simulink model "gm_hdl_model_fixed_vnl"  (R2024a)
settings: Solver=FixedStepDiscrete  StartTime=0.0  StopTime=SIM_TIME  RelTol=1e-3
undefined symbols (not defined in the file or in its folder): a, b, BUFFER_LEN, c, SAMPLING_FREQ, signal_1
libraries: hdlsllib x41, simulink x16, dspsigops x15, simulink_extras x5, dsphdlxfrm2 x2, dspsrcs4 x1
(part 1 of 3)
settings Model: SimulationMode=accelerator  Creator=Jan Rosa  LastModifiedBy=Jan Rosa
settings OptimizationCC: BlockReduction=off  ConditionallyExecuteInputs=off  DefaultParameterBehavior=Inlined  InheritOutputTypeSmallerThanSingle=on
settings DebuggingCC: SignalRangeChecking=warning  AlgebraicLoopMsg=error  SolverPrmCheckMsg=warning  InheritedTsInSrcMsg=none  SingleTaskRateTransMsg=error  UnderSpecifiedDataTypeMsg=warning  UnconnectedInputMsg=error  UnconnectedOutputMsg=error  UnconnectedLineMsg=error  ModelReferenceVersionMismatchMessage=warning  ModelReferenceIOMismatchMessage=warning  ModelReferenceNoExplicitFinalValueMsg=warning  StateNameClashWarn=warning
settings HardwareCC: ProdBitPerPointer=32  ProdBitPerSizeT=32  ProdBitPerPtrDiffT=32  ProdLargestAtomicFloat=None  ProdIntDivRoundTo=Undefined  ProdEndianess=Unspecified  ProdWordSize=32  ProdHWDeviceType=ASIC/FPGA->ASIC/FPGA  TargetBitPerPointer=64  TargetBitPerSizeT=64  TargetBitPerPtrDiffT=64  TargetLongLongMode=on  TargetIntDivRoundTo=Zero  TargetEndianess=LittleEndian  TargetWordSize=64  TargetHWDeviceType=Custom Processor->MATLAB Host Computer  ProdEqTarget=off
settings ModelReferenceCC: EnableRefExpFcnMdlSchedulingChecks=on  EnableParallelModelReferenceBuilds=on

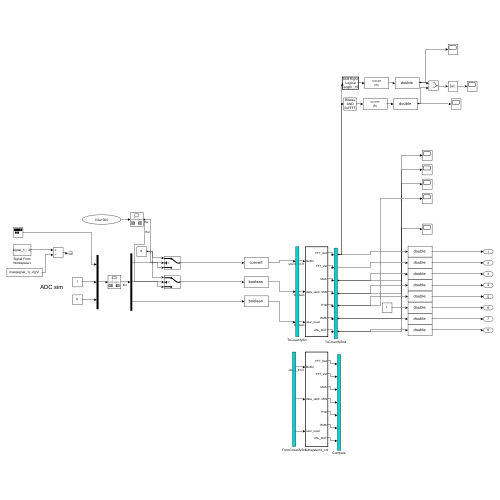
[thumbnail: Simulink's stored preview of the top-level diagram]
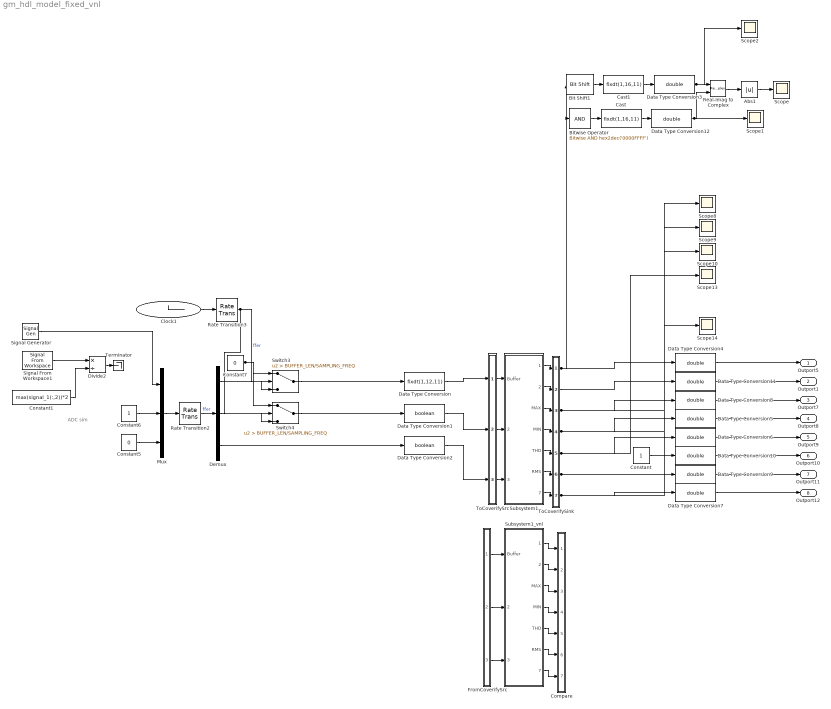
== system gm_hdl_model_fixed_vnl ==
  note: ADC sim
  Abs1 : Abs  SaturateOnIntegerOverflow=off
  Bit Shift1 : hdlsllib/Logic and Bit Operations/Bit Shift  mode=Shift Right Logical  N=16
  Bitwise Operator : simulink/Logic and Bit Operations/Bitwise Operator  logicop=AND  UseBitMask=on  BitMask=hex2dec('0000FFFF')  BitMaskRealWorld=Stored Integer
  Cast : DataTypeConversion  OutDataTypeStr=fixdt(1,16,11)  ConvertRealWorld=Stored Integer (SI)  SaturateOnIntegerOverflow=off  RndMeth=Floor
  Cast1 : DataTypeConversion  OutDataTypeStr=fixdt(1,16,11)  ConvertRealWorld=Stored Integer (SI)  SaturateOnIntegerOverflow=off  RndMeth=Floor
  Clock1 : Clock
  Compare : Subsystem
      mask Display: disp('')
  Constant : Constant
  Constant1 : Constant  Value=max(signal_1(:,2))*2
  Constant5 : Constant  Value=0
  Constant6 : Constant
  Constant7 : Constant  Value=0  SampleTime=1/SAMPLING_FREQ
  Data Type Conversion : DataTypeConversion  OutDataTypeStr=fixdt(1,12,11)  SaturateOnIntegerOverflow=off  RndMeth=Floor  LockScale=on
  Data Type Conversion1 : DataTypeConversion  OutDataTypeStr=boolean  SaturateOnIntegerOverflow=off  RndMeth=Floor  LockScale=on
  Data Type Conversion{3..12} (10 alike) : DataTypeConversion  OutDataTypeStr=double  SaturateOnIntegerOverflow=off  RndMeth=Floor
  Data Type Conversion2 : DataTypeConversion  OutDataTypeStr=boolean  SaturateOnIntegerOverflow=off  RndMeth=Floor  LockScale=on
  Demux : Demux  Outputs=3
  Divide2 : Product  Inputs=*/
  FromCoverifySrc : Subsystem
      mask Display: disp('')
  Mux : Mux  Inputs=3
  Rate Transition2 : RateTransition  Integrity=off  Deterministic=off  OutPortSampleTime=1/SAMPLING_FREQ
  Rate Transition3 : RateTransition  Integrity=off  Deterministic=off  OutPortSampleTime=1/SAMPLING_FREQ
  Real-Imag to Complex : RealImagToComplex
  Scope{,1..2,8..10,13..14} (8 alike) : Scope
  Signal Generator : SignalGenerator  WaveForm=square  Amplitude=0.49999  Frequency=SAMPLING_FREQ/(16*16)
  Signal From Workspace1 : dspsrcs4/Signal From Workspace  X=signal_1(:, 2)  Ts=signal_1(2, 1)  nsamps=1  OutputAfterFinalValue=Cyclic repetition  ignoreOrWarnInputAndFrameLengths=off  OutputFrames=off
  Subsystem1 : Subsystem  TreatAsAtomicUnit=on
  Subsystem1_vnl : Subsystem  TreatAsAtomicUnit=on
  Switch3 : Switch  Criteria=u2 > Threshold  Threshold=BUFFER_LEN/SAMPLING_FREQ  SaturateOnIntegerOverflow=off  InputSameDT=off
  Switch4 : Switch  Criteria=u2 > Threshold  Threshold=BUFFER_LEN/SAMPLING_FREQ  SaturateOnIntegerOverflow=off  InputSameDT=off
  Terminator : Terminator
  ToCoverifySink : Subsystem
      mask Display: disp('')
  ToCoverifySrc : Subsystem
      mask Display: disp('')
  Outport5 : Outport
  Outport1 : Outport  Port=2
  Outport7 : Outport  Port=3
  Outport8 : Outport  Port=4
  Outport9 : Outport  Port=5
  Outport10 : Outport  Port=6
  Outport11 : Outport  Port=7
  Outport12 : Outport  Port=8
  wires:
  Switch4/1 -> Data Type Conversion1/1
  Constant7/1 -> Switch4/1, Switch3/1
  Rate Transition3/1 -> Switch4/2, Switch3/2  "ffer"
  Demux/2 -> Switch4/3
  Clock1/1 -> Rate Transition3/1
  Demux/3 -> Data Type Conversion2/1
  Switch3/1 -> Data Type Conversion/1
  Demux/1 -> Switch3/3
  Mux/1 -> Rate Transition2/1
  Abs1/1 -> Scope/1
  Rate Transition2/1 -> Demux/1  "ffer"
  Constant5/1 -> Mux/3
  Signal From Workspace1/1 -> Divide2/1
  Constant6/1 -> Mux/2
  Constant1/1 -> Divide2/2
  Data Type Conversion4/1 -> Outport5/1
  Data Type Conversion8/1 -> Outport7/1
  Data Type Conversion5/1 -> Outport8/1
  Data Type Conversion6/1 -> Outport9/1
  Data Type Conversion10/1 -> Outport10/1
  Data Type Conversion7/1 -> Outport12/1
  Data Type Conversion9/1 -> Outport11/1
  Data Type Conversion11/1 -> Outport1/1
  Data Type Conversion3/1 -> Scope2/1, Real-Imag to Complex/1
  Real-Imag to Complex/1 -> Abs1/1
  Signal Generator/1 -> Mux/1
  Bit Shift1/1 -> Cast1/1
  Bitwise Operator/1 -> Cast/1
  Data Type Conversion12/1 -> Scope1/1, Real-Imag to Complex/2
  Cast/1 -> Data Type Conversion12/1
  Cast1/1 -> Data Type Conversion3/1
  Constant/1 -> Data Type Conversion10/1
  Divide2/1 -> Terminator/1
  ToCoverifySrc/1(out1) -> Subsystem1/1(Buffer)
  ToCoverifySrc/2(out2) -> Subsystem1/2(data_valid)
  ToCoverifySrc/3(out3) -> Subsystem1/3(user_reset)
  Subsystem1/1(FFT_Dat) -> ToCoverifySink/1(in1)
  Subsystem1/2(FFT_Val) -> ToCoverifySink/2(in2)
  Subsystem1/3(MAX) -> ToCoverifySink/3(in3)
  Subsystem1/4(MIN) -> ToCoverifySink/4(in4)
  Subsystem1/5(THD) -> ToCoverifySink/5(in5)
  Subsystem1/6(RMS) -> ToCoverifySink/6(in6)
  Subsystem1/7(VAL_OUT) -> ToCoverifySink/7(in7)
  Data Type Conversion/1 -> ToCoverifySrc/1(in1)
  Data Type Conversion1/1 -> ToCoverifySrc/2(in2)
  Data Type Conversion2/1 -> ToCoverifySrc/3(in3)
  ToCoverifySink/1(out1) -> Bit Shift1/1, Bitwise Operator/1, Data Type Conversion4/1
  ToCoverifySink/2(out2) -> Data Type Conversion11/1
  ToCoverifySink/3(out3) -> Scope10/1, Data Type Conversion8/1
  ToCoverifySink/4(out4) -> Scope9/1, Data Type Conversion5/1
  ToCoverifySink/5(out5) -> Scope13/1, Data Type Conversion6/1
  ToCoverifySink/6(out6) -> Scope8/1, Data Type Conversion9/1
  ToCoverifySink/7(out7) -> Scope14/1, Data Type Conversion7/1
  FromCoverifySrc/1(out1) -> Subsystem1_vnl/1(Buffer)
  FromCoverifySrc/2(out2) -> Subsystem1_vnl/2(data_valid)
  FromCoverifySrc/3(out3) -> Subsystem1_vnl/3(user_reset)
  Subsystem1_vnl/1(FFT_Dat) -> Compare/1(in1)
  Subsystem1_vnl/2(FFT_Val) -> Compare/2(in2)
  Subsystem1_vnl/3(MAX) -> Compare/3(in3)
  Subsystem1_vnl/4(MIN) -> Compare/4(in4)
  Subsystem1_vnl/5(THD) -> Compare/5(in5)
  Subsystem1_vnl/6(RMS) -> Compare/6(in6)
  Subsystem1_vnl/7(VAL_OUT) -> Compare/7(in7)

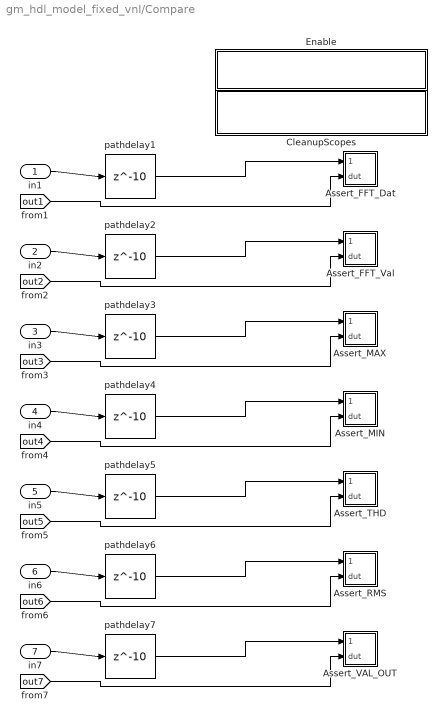
== system gm_hdl_model_fixed_vnl/Compare ==
  in1 : Inport
  in2 : Inport  Port=2
  in3 : Inport  Port=3
  in4 : Inport  Port=4
  in5 : Inport  Port=5
  in6 : Inport  Port=6
  in7 : Inport  Port=7
  Assert_FFT_Dat : Subsystem
      settings: LibrarySourceBlock=hdlmdlgenlib/AssertEqIDC
  Assert_FFT_Val : Subsystem
      settings: LibrarySourceBlock=hdlmdlgenlib/AssertEqIDC
  Assert_MAX : Subsystem
      settings: LibrarySourceBlock=hdlmdlgenlib/AssertEqIDC
  Assert_MIN : Subsystem
      settings: LibrarySourceBlock=hdlmdlgenlib/AssertEqIDC
  Assert_RMS : Subsystem
      settings: LibrarySourceBlock=hdlmdlgenlib/AssertEqIDC
  Assert_THD : Subsystem
      settings: LibrarySourceBlock=hdlmdlgenlib/AssertEqIDC
  Assert_VAL_OUT : Subsystem
      settings: LibrarySourceBlock=hdlmdlgenlib/AssertEqIDC
  CleanupScopes : Subsystem
      settings: OpenFcn=|
      | blkName = gcb; %self block
      | idx = regexp(blkName, '/CleanupScopes$', 'once');
      | blkParent = blkName(1:idx-1);
      | blks=find_system(blkParent, 'LookUnderMasks', 'all','blocktype', 'Scope');
      | for itr = 1:length(blks)
      | 	 hScopeCfg = get_param(blks{itr},'ScopeConfiguration');
      | 	 hScopeCfg.Visible = ~ hScopeCfg.Visible;
      | end
      | drawnow;
      mask Display: fprintf(message('hdlcoder:cosim:vnl_dblclick').getString());
  Enable : Subsystem
      settings: OpenFcn=|
      | blkName = gcb;
      | idx = regexp(blkName, '/Enable$', 'once');
      | blkParent = blkName(1:idx-1);
      | blks=find_system(blkParent, 'LookUnderMasks', 'all','blocktype', 'Assertion');
      | e = get_param(blks{1}, 'Enabled');
      | if strcmp(e, 'on'), f= 'off';, else, f = 'on';, end
      | for ii=1:length(blks), set_param(blks{ii}, 'Enabled', f);, end
      | set_param(gcb, 'MaskDisplay',['fprintf(message(''hdlcoder:cosim:vnl_dblclick_assertions'',','''',upper(e),'''',').getString())']);
      mask Display: fprintf(message('hdlcoder:cosim:vnl_dblclick_assertions','OFF').getString());
  pathdelay{1..7} (7 alike) : Delay  DelayLength=10
  wires:
  in1/1 -> pathdelay1/1
  pathdelay1/1 -> Assert_FFT_Dat/1(cosim)
  [out1] -> Assert_FFT_Dat/2(dut)
  in2/1 -> pathdelay2/1
  pathdelay2/1 -> Assert_FFT_Val/1(cosim)
  [out2] -> Assert_FFT_Val/2(dut)
  in3/1 -> pathdelay3/1
  pathdelay3/1 -> Assert_MAX/1(cosim)
  [out3] -> Assert_MAX/2(dut)
  in4/1 -> pathdelay4/1
  pathdelay4/1 -> Assert_MIN/1(cosim)
  [out4] -> Assert_MIN/2(dut)
  in5/1 -> pathdelay5/1
  pathdelay5/1 -> Assert_THD/1(cosim)
  [out5] -> Assert_THD/2(dut)
  in6/1 -> pathdelay6/1
  pathdelay6/1 -> Assert_RMS/1(cosim)
  [out6] -> Assert_RMS/2(dut)
  in7/1 -> pathdelay7/1
  pathdelay7/1 -> Assert_VAL_OUT/1(cosim)
  [out7] -> Assert_VAL_OUT/2(dut)

== system gm_hdl_model_fixed_vnl/FromCoverifySrc ==
  out1 : Outport
  out2 : Outport  Port=2
  out3 : Outport  Port=3
  wires:
  [in1] -> out1/1
  [in2] -> out2/1
  [in3] -> out3/1

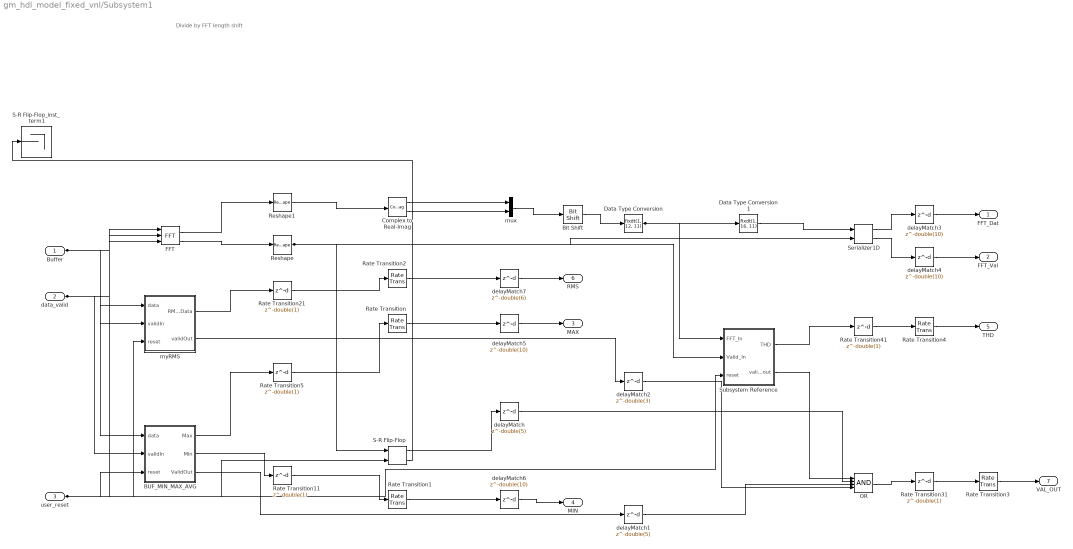
== system gm_hdl_model_fixed_vnl/Subsystem1 ==
  note: Divide by FFT length shift
  Buffer : Inport  OutDataTypeStr=fixdt(1, 12, 11)  PortDimensions=1  SampleTime=1e-08
  data_valid : Inport  Port=2  OutDataTypeStr=boolean  PortDimensions=1  SampleTime=1e-08
  user_reset : Inport  Port=3  OutDataTypeStr=boolean  PortDimensions=1  SampleTime=1e-08
  BUF_MIN_MAX_AVG : Subsystem
  Bit Shift : hdlsllib/Logic and Bit Operations/Bit Shift  mode=Shift Right Arithmetic  N=double(11)
  Complex to Real-Imag : ComplexToRealImag  SampleTime=1e-08
  Data Type Conversion : DataTypeConversion  OutDataTypeStr=fixdt(1, 12, 11)  SampleTime=1e-08  SaturateOnIntegerOverflow=off  RndMeth=Floor
  Data Type Conversion1 : DataTypeConversion  OutDataTypeStr=fixdt(1, 16, 11)  SampleTime=1e-08  SaturateOnIntegerOverflow=off  RndMeth=Floor
  FFT : dsphdlxfrm2/FFT  Architecture=Streaming Radix 2^2  FFTLengthSource=Property  FFTLength=BUFFER_LEN  FFTLengthMax=1024  ComplexMultiplication=Use 4 multipliers and 2 adders  BitReversedOutput=off  BitReversedInput=off  Normalize=off  SimulateUsing=Code generation  RoundingMethod=Floor  ResetInputPort=on  StartOutputPort=off  EndOutputPort=off
  OR : Logic  Inputs=4  AllPortsSameDT=off  OutDataTypeStr=boolean  SampleTime=1e-08
  Rate Transition : RateTransition  Integrity=off  Deterministic=off  InitialCondition="fi(0,0,16,16,\"hex\",\"0000\")"  OutPortSampleTimeOpt=Multiple of input port sample time  OutPortSampleTimeMultiple=1/2
  Rate Transition1 : RateTransition  Integrity=off  Deterministic=off  InitialCondition="fi(0,1,16,15,\"hex\",\"0000\")"  OutPortSampleTimeOpt=Multiple of input port sample time  OutPortSampleTimeMultiple=1/2
  Rate Transition{5,11,21,31,41} (5 alike) : Delay  DelayLength=double(1)  InitialCondition=0  SampleTime=1e-08
  Rate Transition2 : RateTransition  Integrity=off  Deterministic=off  InitialCondition="fi(0,0,16,7,\"hex\",\"0000\")"  OutPortSampleTimeOpt=Multiple of input port sample time  OutPortSampleTimeMultiple=1/2
  Rate Transition3 : RateTransition  Integrity=off  Deterministic=off  OutPortSampleTimeOpt=Multiple of input port sample time  OutPortSampleTimeMultiple=1/2
  Rate Transition4 : RateTransition  Integrity=off  Deterministic=off  InitialCondition="fi(0,1,18,10,\"hex\",\"00000\")"  OutPortSampleTimeOpt=Multiple of input port sample time  OutPortSampleTimeMultiple=1/2
  Reshape : Reshape
  Reshape1 : Reshape
  S-R Flip-Flop : simulink_extras/Flip Flops/S-R Flip-Flop  initial_condition=0
  S-R Flip-Flop_inst_term1 : Terminator
  Serializer1D : hdlsllib/HDL Operations/Serializer1D  Ratio=2  IdleCycles=0  validIn=on  startOut=off  validOut=on  inputDataDimensions=2  inputSampleTime=1e-08  inputSignalType=real
  Subsystem Reference : Subsystem
  delayMatch : Delay  DelayLength=double(5)  InitialCondition=0  SampleTime=1e-08
  delayMatch1 : Delay  DelayLength=double(5)  InitialCondition=0  SampleTime=1e-08
  delayMatch2 : Delay  DelayLength=double(3)  InitialCondition=0  SampleTime=1e-08
  delayMatch{3..6} (4 alike) : Delay  DelayLength=double(10)  InitialCondition=0  SampleTime=5e-09
  delayMatch7 : Delay  DelayLength=double(6)  InitialCondition=0  SampleTime=5e-09
  mux : Mux  Inputs=2
  myRMS : Subsystem
  FFT_Dat : Outport  SampleTime=5e-09
  FFT_Val : Outport  Port=2  SampleTime=5e-09
  MAX : Outport  Port=3  SampleTime=5e-09
  MIN : Outport  Port=4  SampleTime=5e-09
  THD : Outport  Port=5  SampleTime=5e-09
  RMS : Outport  Port=6  SampleTime=5e-09
  VAL_OUT : Outport  Port=7  SampleTime=5e-09
  wires:
  Rate Transition2/1 -> delayMatch7/1
  Rate Transition1/1 -> delayMatch6/1
  Rate Transition/1 -> delayMatch5/1
  Serializer1D/2 -> delayMatch4/1
  Serializer1D/1 -> delayMatch3/1
  myRMS/2(validOut) -> delayMatch2/1
  BUF_MIN_MAX_AVG/3(ValidOut) -> delayMatch1/1
  S-R Flip-Flop/1 -> delayMatch/1
  OR/1 -> Rate Transition31/1
  Data Type Conversion1/1 -> Serializer1D/1
  Bit Shift/1 -> Data Type Conversion/1
  mux/1 -> Bit Shift/1
  Complex to Real-Imag/2 -> mux/2
  Complex to Real-Imag/1 -> mux/1
  Reshape1/1 -> Complex to Real-Imag/1
  S-R Flip-Flop/2 -> S-R Flip-Flop_inst_term1/1
  Rate Transition41/1 -> Rate Transition4/1
  Rate Transition31/1 -> Rate Transition3/1
  Rate Transition21/1 -> Rate Transition2/1
  Rate Transition11/1 -> Rate Transition1/1
  Rate Transition5/1 -> Rate Transition/1
  delayMatch/1 -> OR/2
  delayMatch4/1 -> FFT_Val/1
  Rate Transition4/1 -> THD/1
  Rate Transition3/1 -> VAL_OUT/1
  delayMatch7/1 -> RMS/1
  delayMatch6/1 -> MIN/1
  delayMatch5/1 -> MAX/1
  delayMatch2/1 -> OR/4
  myRMS/1(RMS_Data) -> Rate Transition21/1
  Subsystem Reference/2(valid_out) -> OR/1
  Subsystem Reference/1(THD) -> Rate Transition41/1
  delayMatch3/1 -> FFT_Dat/1
  Reshape/1 -> S-R Flip-Flop/1, Serializer1D/2, Subsystem Reference/2(Valid_In)
  FFT/2 -> Reshape/1
  FFT/1 -> Reshape1/1
  Data Type Conversion/1 -> Data Type Conversion1/1, Subsystem Reference/1(FFT_In)
  delayMatch1/1 -> OR/3
  BUF_MIN_MAX_AVG/2(Min) -> Rate Transition11/1
  BUF_MIN_MAX_AVG/1(Max) -> Rate Transition5/1
  user_reset/1 -> FFT/3, S-R Flip-Flop/2, Subsystem Reference/3(reset), BUF_MIN_MAX_AVG/3(reset), myRMS/3(reset)
  data_valid/1 -> FFT/2, myRMS/2(validIn), BUF_MIN_MAX_AVG/2(validIn)
  Buffer/1 -> FFT/1, myRMS/1(data), BUF_MIN_MAX_AVG/1(data)

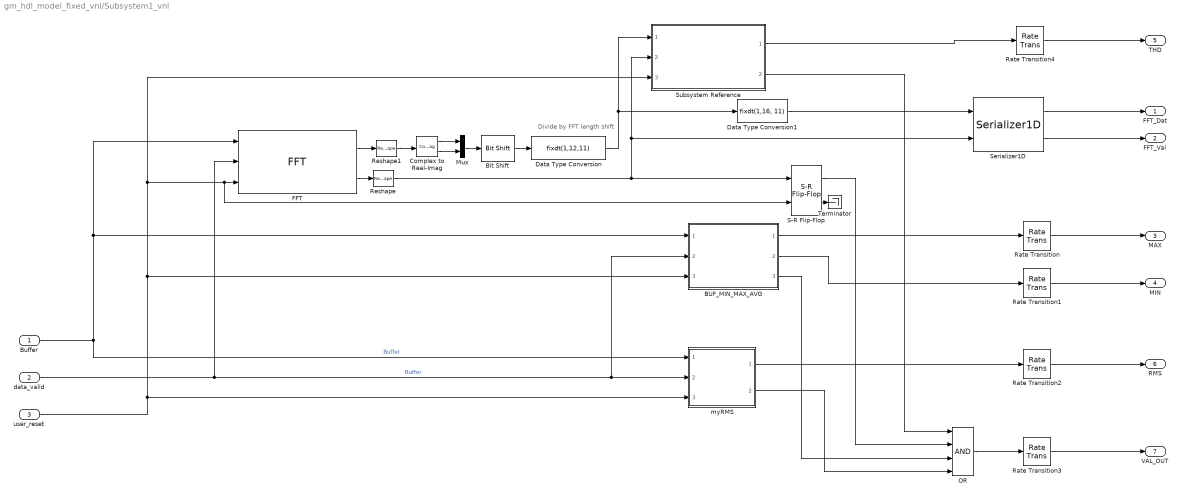
== system gm_hdl_model_fixed_vnl/Subsystem1_vnl ==
  note: Divide by FFT length shift
  Buffer : Inport  OutDataTypeStr=fixdt(1,12,11)
  data_valid : Inport  Port=2
  user_reset : Inport  Port=3
  BUF_MIN_MAX_AVG : Subsystem  TreatAsAtomicUnit=on  ReferencedSubsystem=BUF_MIN_MAX_AVG_fixed
  Bit Shift : hdlsllib/Logic and Bit Operations/Bit Shift  mode=Shift Right Arithmetic  N=log2(BUFFER_LEN)
  Complex to Real-Imag : ComplexToRealImag
  Data Type Conversion : DataTypeConversion  OutDataTypeStr=fixdt(1,12,11)  SaturateOnIntegerOverflow=off  RndMeth=Floor
  Data Type Conversion1 : DataTypeConversion  OutDataTypeStr=fixdt(1,16, 11)  SaturateOnIntegerOverflow=off  RndMeth=Floor
  FFT : dsphdlxfrm2/FFT  Architecture=Streaming Radix 2^2  FFTLengthSource=Property  FFTLength=BUFFER_LEN  FFTLengthMax=1024  ComplexMultiplication=Use 4 multipliers and 2 adders  BitReversedOutput=off  BitReversedInput=off  Normalize=off  SimulateUsing=Code generation  RoundingMethod=Floor  ResetInputPort=on  StartOutputPort=off  EndOutputPort=off
  Mux : Mux  Inputs=2
  OR : Logic  Inputs=4  IconShape=distinctive  AllPortsSameDT=off  OutDataTypeStr=boolean
  Rate Transition{,1..4} (5 alike) : RateTransition  OutPortSampleTime=1/(2*SAMPLING_FREQ)
  Reshape : Reshape  OutputDimensionality=Customize  OutputDimensions=[1]
  Reshape1 : Reshape  OutputDimensionality=Customize  OutputDimensions=[1]
  S-R Flip-Flop : simulink_extras/Flip Flops/S-R Flip-Flop  initial_condition=0
  Serializer1D : hdlsllib/HDL Operations/Serializer1D  Ratio=2  IdleCycles=0  validIn=on  startOut=off  validOut=on  inputDataDimensions=-1  inputSampleTime=-1  inputSignalType=auto
  Subsystem Reference : Subsystem  TreatAsAtomicUnit=on  ReferencedSubsystem=myTHD_fixed
  Terminator : Terminator
  myRMS : Subsystem  TreatAsAtomicUnit=on  ReferencedSubsystem=myRMS_fixed
  FFT_Dat : Outport
  FFT_Val : Outport  Port=2
  MAX : Outport  Port=3
  MIN : Outport  Port=4
  THD : Outport  Port=5
  RMS : Outport  Port=6
  VAL_OUT : Outport  Port=7
  wires:
  Rate Transition4/1 -> THD/1
  Rate Transition3/1 -> VAL_OUT/1
  Rate Transition2/1 -> RMS/1
  Rate Transition1/1 -> MIN/1
  Rate Transition/1 -> MAX/1
  Serializer1D/2 -> FFT_Val/1
  Complex to Real-Imag/1 -> Mux/1
  Complex to Real-Imag/2 -> Mux/2
  Mux/1 -> Bit Shift/1
  Reshape1/1 -> Complex to Real-Imag/1
  Reshape/1 -> Subsystem Reference/2, Serializer1D/2, S-R Flip-Flop/1
  FFT/2 -> Reshape/1
  S-R Flip-Flop/2 -> Terminator/1
  Serializer1D/1 -> FFT_Dat/1
  Data Type Conversion1/1 -> Serializer1D/1
  Data Type Conversion/1 -> Data Type Conversion1/1, Subsystem Reference/1
  S-R Flip-Flop/1 -> OR/2
  FFT/1 -> Reshape1/1
  Bit Shift/1 -> Data Type Conversion/1
  user_reset/1 -> Subsystem Reference/3, S-R Flip-Flop/2, FFT/3, BUF_MIN_MAX_AVG/3, myRMS/3
  Subsystem Reference/2 -> OR/1
  Subsystem Reference/1 -> Rate Transition4/1
  data_valid/1 -> myRMS/2, BUF_MIN_MAX_AVG/2, FFT/2  "Buffer"
  Buffer/1 -> myRMS/1, FFT/1, BUF_MIN_MAX_AVG/1  "Buffer"
  myRMS/2 -> OR/4
  myRMS/1 -> Rate Transition2/1
  BUF_MIN_MAX_AVG/3 -> OR/3
  BUF_MIN_MAX_AVG/2 -> Rate Transition1/1
  BUF_MIN_MAX_AVG/1 -> Rate Transition/1
  OR/1 -> Rate Transition3/1

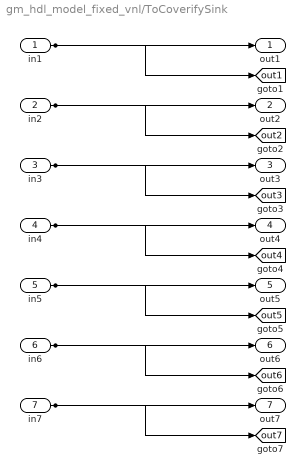
== system gm_hdl_model_fixed_vnl/ToCoverifySink ==
  in1 : Inport
  in2 : Inport  Port=2
  in3 : Inport  Port=3
  in4 : Inport  Port=4
  in5 : Inport  Port=5
  in6 : Inport  Port=6
  in7 : Inport  Port=7
  out1 : Outport
  out2 : Outport  Port=2
  out3 : Outport  Port=3
  out4 : Outport  Port=4
  out5 : Outport  Port=5
  out6 : Outport  Port=6
  out7 : Outport  Port=7
  tag scope: out1=global, out2=global, out3=global, out4=global, out5=global, out6=global, out7=global
  wires:
  in1/1 -> out1/1, [out1]
  in2/1 -> out2/1, [out2]
  in3/1 -> out3/1, [out3]
  in4/1 -> out4/1, [out4]
  in5/1 -> out5/1, [out5]
  in6/1 -> out6/1, [out6]
  in7/1 -> out7/1, [out7]

== system gm_hdl_model_fixed_vnl/ToCoverifySrc ==
  in1 : Inport
  in2 : Inport  Port=2
  in3 : Inport  Port=3
  out1 : Outport
  out2 : Outport  Port=2
  out3 : Outport  Port=3
  tag scope: in1=global, in2=global, in3=global
  wires:
  in1/1 -> out1/1, [in1]
  in2/1 -> out2/1, [in2]
  in3/1 -> out3/1, [in3]

== system gm_hdl_model_fixed_vnl/Compare/Assert_FFT_Dat ==
  cosim : Inport
  dut : Inport  Port=2
  AssertEq : Assertion  StopWhenAssertionFail=off
  Compare To Zero : simulink/Logic and Bit Operations/Compare To Zero  relop===  OutDataTypeStr=boolean
  Constant1 : Constant  Value=0  OutDataTypeStr=Inherit: Inherit via back propagation  SampleTime=-1
  Counter : simulink/Sources/Counter Free-Running  NumBits=32  tsamp=-1
  IgnoreCycles : Constant  Value=10  OutDataTypeStr=Inherit: Inherit via back propagation  SampleTime=-1
  Relational Operator : RelationalOperator  Operator=<  OutDataTypeStr=boolean  InputSameDT=off
  Relational Operator1 : RelationalOperator  Operator===  OutDataTypeStr=boolean  InputSameDT=off
  Switch : Switch  Criteria=u2 ~= 0  SaturateOnIntegerOverflow=off  InputSameDT=off
  Switch1 : Switch  Criteria=u2 ~= 0  SaturateOnIntegerOverflow=off  InputSameDT=off
  compare: FFT_Dat : Scope  NumInputPorts=3
  wires:
  Compare To Zero/1 -> compare: FFT_Dat/3  "err"
  Relational Operator1/1 -> Compare To Zero/1, AssertEq/1
  Switch1/1 -> compare: FFT_Dat/1, Relational Operator1/1
  Switch/1 -> compare: FFT_Dat/2, Relational Operator1/2
  Constant1/1 -> Switch/1, Switch1/1
  Relational Operator/1 -> Switch/2, Switch1/2
  cosim/1 -> Switch1/3  "cosim"
  dut/1 -> Switch/3  "dut ref"
  Counter/1 -> Relational Operator/1
  IgnoreCycles/1 -> Relational Operator/2

== system gm_hdl_model_fixed_vnl/Compare/Assert_FFT_Val ==
  cosim : Inport
  dut : Inport  Port=2
  AssertEq : Assertion  StopWhenAssertionFail=off
  Compare To Zero : simulink/Logic and Bit Operations/Compare To Zero  relop===  OutDataTypeStr=boolean
  Constant1 : Constant  Value=0  OutDataTypeStr=Inherit: Inherit via back propagation  SampleTime=-1
  Counter : simulink/Sources/Counter Free-Running  NumBits=32  tsamp=-1
  IgnoreCycles : Constant  Value=10  OutDataTypeStr=Inherit: Inherit via back propagation  SampleTime=-1
  Relational Operator : RelationalOperator  Operator=<  OutDataTypeStr=boolean  InputSameDT=off
  Relational Operator1 : RelationalOperator  Operator===  OutDataTypeStr=boolean  InputSameDT=off
  Switch : Switch  Criteria=u2 ~= 0  SaturateOnIntegerOverflow=off  InputSameDT=off
  Switch1 : Switch  Criteria=u2 ~= 0  SaturateOnIntegerOverflow=off  InputSameDT=off
  compare: FFT_Val : Scope  NumInputPorts=3
  wires:
  Compare To Zero/1 -> compare: FFT_Val/3  "err"
  Relational Operator1/1 -> Compare To Zero/1, AssertEq/1
  Switch1/1 -> compare: FFT_Val/1, Relational Operator1/1
  Switch/1 -> compare: FFT_Val/2, Relational Operator1/2
  Constant1/1 -> Switch/1, Switch1/1
  Relational Operator/1 -> Switch/2, Switch1/2
  cosim/1 -> Switch1/3  "cosim"
  dut/1 -> Switch/3  "dut ref"
  Counter/1 -> Relational Operator/1
  IgnoreCycles/1 -> Relational Operator/2

== system gm_hdl_model_fixed_vnl/Compare/Assert_MAX ==
  cosim : Inport
  dut : Inport  Port=2
  AssertEq : Assertion  StopWhenAssertionFail=off
  Compare To Zero : simulink/Logic and Bit Operations/Compare To Zero  relop===  OutDataTypeStr=boolean
  Constant1 : Constant  Value=0  OutDataTypeStr=Inherit: Inherit via back propagation  SampleTime=-1
  Counter : simulink/Sources/Counter Free-Running  NumBits=32  tsamp=-1
  IgnoreCycles : Constant  Value=10  OutDataTypeStr=Inherit: Inherit via back propagation  SampleTime=-1
  Relational Operator : RelationalOperator  Operator=<  OutDataTypeStr=boolean  InputSameDT=off
  Relational Operator1 : RelationalOperator  Operator===  OutDataTypeStr=boolean  InputSameDT=off
  Switch : Switch  Criteria=u2 ~= 0  SaturateOnIntegerOverflow=off  InputSameDT=off
  Switch1 : Switch  Criteria=u2 ~= 0  SaturateOnIntegerOverflow=off  InputSameDT=off
  compare: MAX : Scope  NumInputPorts=3
  wires:
  Compare To Zero/1 -> compare: MAX/3  "err"
  Relational Operator1/1 -> Compare To Zero/1, AssertEq/1
  Switch1/1 -> compare: MAX/1, Relational Operator1/1
  Switch/1 -> compare: MAX/2, Relational Operator1/2
  Constant1/1 -> Switch/1, Switch1/1
  Relational Operator/1 -> Switch/2, Switch1/2
  cosim/1 -> Switch1/3  "cosim"
  dut/1 -> Switch/3  "dut ref"
  Counter/1 -> Relational Operator/1
  IgnoreCycles/1 -> Relational Operator/2

== system gm_hdl_model_fixed_vnl/Compare/Assert_MIN ==
  cosim : Inport
  dut : Inport  Port=2
  AssertEq : Assertion  StopWhenAssertionFail=off
  Compare To Zero : simulink/Logic and Bit Operations/Compare To Zero  relop===  OutDataTypeStr=boolean
  Constant1 : Constant  Value=0  OutDataTypeStr=Inherit: Inherit via back propagation  SampleTime=-1
  Counter : simulink/Sources/Counter Free-Running  NumBits=32  tsamp=-1
  IgnoreCycles : Constant  Value=10  OutDataTypeStr=Inherit: Inherit via back propagation  SampleTime=-1
  Relational Operator : RelationalOperator  Operator=<  OutDataTypeStr=boolean  InputSameDT=off
  Relational Operator1 : RelationalOperator  Operator===  OutDataTypeStr=boolean  InputSameDT=off
  Switch : Switch  Criteria=u2 ~= 0  SaturateOnIntegerOverflow=off  InputSameDT=off
  Switch1 : Switch  Criteria=u2 ~= 0  SaturateOnIntegerOverflow=off  InputSameDT=off
  compare: MIN : Scope  NumInputPorts=3
  wires:
  Compare To Zero/1 -> compare: MIN/3  "err"
  Relational Operator1/1 -> Compare To Zero/1, AssertEq/1
  Switch1/1 -> compare: MIN/1, Relational Operator1/1
  Switch/1 -> compare: MIN/2, Relational Operator1/2
  Constant1/1 -> Switch/1, Switch1/1
  Relational Operator/1 -> Switch/2, Switch1/2
  cosim/1 -> Switch1/3  "cosim"
  dut/1 -> Switch/3  "dut ref"
  Counter/1 -> Relational Operator/1
  IgnoreCycles/1 -> Relational Operator/2

== system gm_hdl_model_fixed_vnl/Compare/Assert_RMS ==
  cosim : Inport
  dut : Inport  Port=2
  AssertEq : Assertion  StopWhenAssertionFail=off
  Compare To Zero : simulink/Logic and Bit Operations/Compare To Zero  relop===  OutDataTypeStr=boolean
  Constant1 : Constant  Value=0  OutDataTypeStr=Inherit: Inherit via back propagation  SampleTime=-1
  Counter : simulink/Sources/Counter Free-Running  NumBits=32  tsamp=-1
  IgnoreCycles : Constant  Value=10  OutDataTypeStr=Inherit: Inherit via back propagation  SampleTime=-1
  Relational Operator : RelationalOperator  Operator=<  OutDataTypeStr=boolean  InputSameDT=off
  Relational Operator1 : RelationalOperator  Operator===  OutDataTypeStr=boolean  InputSameDT=off
  Switch : Switch  Criteria=u2 ~= 0  SaturateOnIntegerOverflow=off  InputSameDT=off
  Switch1 : Switch  Criteria=u2 ~= 0  SaturateOnIntegerOverflow=off  InputSameDT=off
  compare: RMS : Scope  NumInputPorts=3
  wires:
  Compare To Zero/1 -> compare: RMS/3  "err"
  Relational Operator1/1 -> Compare To Zero/1, AssertEq/1
  Switch1/1 -> compare: RMS/1, Relational Operator1/1
  Switch/1 -> compare: RMS/2, Relational Operator1/2
  Constant1/1 -> Switch/1, Switch1/1
  Relational Operator/1 -> Switch/2, Switch1/2
  cosim/1 -> Switch1/3  "cosim"
  dut/1 -> Switch/3  "dut ref"
  Counter/1 -> Relational Operator/1
  IgnoreCycles/1 -> Relational Operator/2

== system gm_hdl_model_fixed_vnl/Compare/Assert_THD ==
  cosim : Inport
  dut : Inport  Port=2
  AssertEq : Assertion  StopWhenAssertionFail=off
  Compare To Zero : simulink/Logic and Bit Operations/Compare To Zero  relop===  OutDataTypeStr=boolean
  Constant1 : Constant  Value=0  OutDataTypeStr=Inherit: Inherit via back propagation  SampleTime=-1
  Counter : simulink/Sources/Counter Free-Running  NumBits=32  tsamp=-1
  IgnoreCycles : Constant  Value=10  OutDataTypeStr=Inherit: Inherit via back propagation  SampleTime=-1
  Relational Operator : RelationalOperator  Operator=<  OutDataTypeStr=boolean  InputSameDT=off
  Relational Operator1 : RelationalOperator  Operator===  OutDataTypeStr=boolean  InputSameDT=off
  Switch : Switch  Criteria=u2 ~= 0  SaturateOnIntegerOverflow=off  InputSameDT=off
  Switch1 : Switch  Criteria=u2 ~= 0  SaturateOnIntegerOverflow=off  InputSameDT=off
  compare: THD : Scope  NumInputPorts=3
  wires:
  Compare To Zero/1 -> compare: THD/3  "err"
  Relational Operator1/1 -> Compare To Zero/1, AssertEq/1
  Switch1/1 -> compare: THD/1, Relational Operator1/1
  Switch/1 -> compare: THD/2, Relational Operator1/2
  Constant1/1 -> Switch/1, Switch1/1
  Relational Operator/1 -> Switch/2, Switch1/2
  cosim/1 -> Switch1/3  "cosim"
  dut/1 -> Switch/3  "dut ref"
  Counter/1 -> Relational Operator/1
  IgnoreCycles/1 -> Relational Operator/2

== system gm_hdl_model_fixed_vnl/Compare/Assert_VAL_OUT ==
  cosim : Inport
  dut : Inport  Port=2
  AssertEq : Assertion  StopWhenAssertionFail=off
  Compare To Zero : simulink/Logic and Bit Operations/Compare To Zero  relop===  OutDataTypeStr=boolean
  Constant1 : Constant  Value=0  OutDataTypeStr=Inherit: Inherit via back propagation  SampleTime=-1
  Counter : simulink/Sources/Counter Free-Running  NumBits=32  tsamp=-1
  IgnoreCycles : Constant  Value=10  OutDataTypeStr=Inherit: Inherit via back propagation  SampleTime=-1
  Relational Operator : RelationalOperator  Operator=<  OutDataTypeStr=boolean  InputSameDT=off
  Relational Operator1 : RelationalOperator  Operator===  OutDataTypeStr=boolean  InputSameDT=off
  Switch : Switch  Criteria=u2 ~= 0  SaturateOnIntegerOverflow=off  InputSameDT=off
  Switch1 : Switch  Criteria=u2 ~= 0  SaturateOnIntegerOverflow=off  InputSameDT=off
  compare: VAL_OUT : Scope  NumInputPorts=3
  wires:
  Compare To Zero/1 -> compare: VAL_OUT/3  "err"
  Relational Operator1/1 -> Compare To Zero/1, AssertEq/1
  Switch1/1 -> compare: VAL_OUT/1, Relational Operator1/1
  Switch/1 -> compare: VAL_OUT/2, Relational Operator1/2
  Constant1/1 -> Switch/1, Switch1/1
  Relational Operator/1 -> Switch/2, Switch1/2
  cosim/1 -> Switch1/3  "cosim"
  dut/1 -> Switch/3  "dut ref"
  Counter/1 -> Relational Operator/1
  IgnoreCycles/1 -> Relational Operator/2

== system gm_hdl_model_fixed_vnl/Compare/CleanupScopes ==

== system gm_hdl_model_fixed_vnl/Compare/Enable ==

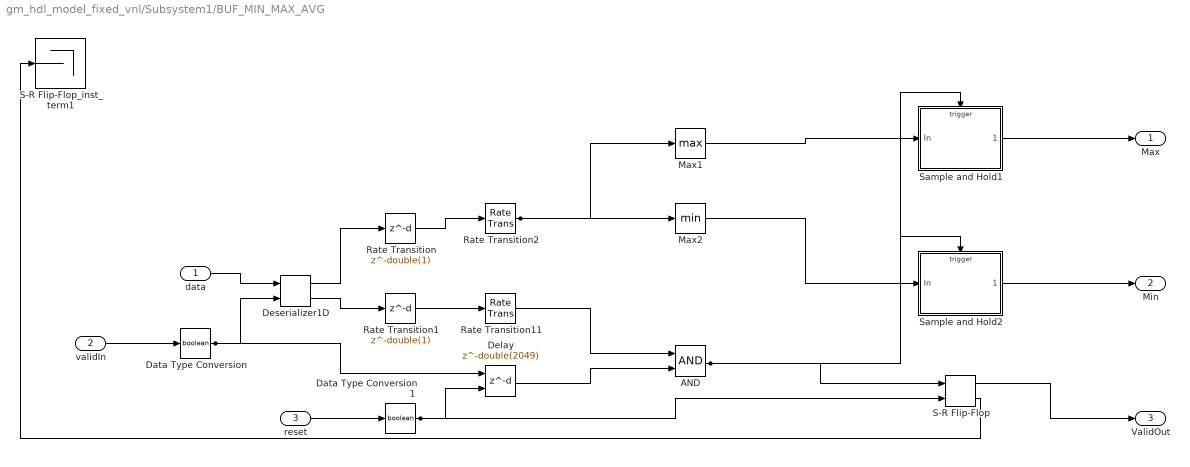
== system gm_hdl_model_fixed_vnl/Subsystem1/BUF_MIN_MAX_AVG ==
  data : Inport  OutDataTypeStr=fixdt(1, 12, 11)  PortDimensions=1  SampleTime=1e-08
  validIn : Inport  Port=2  OutDataTypeStr=boolean  PortDimensions=1  SampleTime=1e-08
  reset : Inport  Port=3  OutDataTypeStr=boolean  PortDimensions=1  SampleTime=1e-08
  AND : Logic  AllPortsSameDT=off  OutDataTypeStr=boolean  SampleTime=1e-08
  Data Type Conversion : DataTypeConversion  OutDataTypeStr=boolean
  Data Type Conversion1 : DataTypeConversion  OutDataTypeStr=boolean
  Delay : Delay  DelayLength=double(2049)  InitialCondition=0  ExternalReset=Level
      settings: InputPortMap=u0,r5
  Deserializer1D : hdlsllib/HDL Operations/Deserializer1D  Ratio=2048  IdleCycles=0  InitialCondition=0  startIn=off  validIn=on  validOut=on  inputDataDimensions=1  inputSampleTime=1e-08  inputSignalType=real
  Max1 : MinMax  Function=max  OutDataTypeStr=fixdt(0,16,16)
  Max2 : MinMax  OutDataTypeStr=fixdt(1,16,15)
  Rate Transition : Delay  DelayLength=double(1)  InitialCondition=0  SampleTime=2.048e-05
  Rate Transition1 : Delay  DelayLength=double(1)  InitialCondition=0  SampleTime=2.048e-05
  Rate Transition11 : RateTransition  Integrity=off  Deterministic=off  OutPortSampleTimeOpt=Multiple of input port sample time  OutPortSampleTimeMultiple=1/2048
  Rate Transition2 : RateTransition  Integrity=off  Deterministic=off  InitialCondition="fi(0,1,12,11,\"hex\",\"000\")"  OutPortSampleTimeOpt=Multiple of input port sample time  OutPortSampleTimeMultiple=1/2048
  S-R Flip-Flop : simulink_extras/Flip Flops/S-R Flip-Flop  initial_condition=0
  S-R Flip-Flop_inst_term1 : Terminator
  Sample and Hold1 : Subsystem  mask(Sample and Hold){trig=Rising edge, initCond=double(0), latchinput=off}
      mask prompts: trig "dsp:DSPSignalOperationsBlockDialog:TriggerType_MP"; initCond "dsp:DSPSignalOperationsBlockDialog:InitialCondition_MP"; latchinput "dsp:DSPSignalOperationsBlockDialog:LatchInput_MP"
      mask help: dsp:DSPSignalOperationsBlockDialog:SampleAndHold_MaskDesc
      mask init:
      | initCond = double(0);
      | latchinput = double(0);
      | s = 'rising';
      | trig = double(1);
      mask Help: eval('blocksethelp');
      mask TypeOptions trig: dsp:DSPSignalOperationsBlockDialog:RisingEdge_MP | dsp:DSPSignalOperationsBlockDialog:FallingEdge_MP | dsp:DSPSignalOperationsBlockDialog:EitherEdge_MP
      mask Display: disp('S/H')
  Sample and Hold2 : Subsystem  mask(Sample and Hold){trig=Rising edge, initCond=double(0), latchinput=off}
      mask prompts: trig "dsp:DSPSignalOperationsBlockDialog:TriggerType_MP"; initCond "dsp:DSPSignalOperationsBlockDialog:InitialCondition_MP"; latchinput "dsp:DSPSignalOperationsBlockDialog:LatchInput_MP"
      mask help: dsp:DSPSignalOperationsBlockDialog:SampleAndHold_MaskDesc
      mask init:
      | initCond = double(0);
      | latchinput = double(0);
      | s = 'rising';
      | trig = double(1);
      mask Help: eval('blocksethelp');
      mask TypeOptions trig: dsp:DSPSignalOperationsBlockDialog:RisingEdge_MP | dsp:DSPSignalOperationsBlockDialog:FallingEdge_MP | dsp:DSPSignalOperationsBlockDialog:EitherEdge_MP
      mask Display: disp('S/H')
  Max : Outport  SampleTime=1e-08
  Min : Outport  Port=2  SampleTime=1e-08
  ValidOut : Outport  Port=3  SampleTime=1e-08
  wires:
  Deserializer1D/1 -> Rate Transition/1
  S-R Flip-Flop/2 -> S-R Flip-Flop_inst_term1/1
  AND/1 -> S-R Flip-Flop/1, Sample and Hold2/Trigger, Sample and Hold1/Trigger
  Data Type Conversion/1 -> Delay/1, Deserializer1D/2
  Rate Transition2/1 -> Max1/1, Max2/1
  Rate Transition11/1 -> AND/1
  Rate Transition/1 -> Rate Transition2/1
  Rate Transition1/1 -> Rate Transition11/1
  Max1/1 -> Sample and Hold1/1(In)
  Max2/1 -> Sample and Hold2/1(In)
  Data Type Conversion1/1 -> S-R Flip-Flop/2, Delay/2
  Deserializer1D/2 -> Rate Transition1/1
  Sample and Hold2/1(" ") -> Min/1
  Sample and Hold1/1(" ") -> Max/1
  S-R Flip-Flop/1 -> ValidOut/1
  Delay/1 -> AND/2
  reset/1 -> Data Type Conversion1/1
  validIn/1 -> Data Type Conversion/1
  data/1 -> Deserializer1D/1

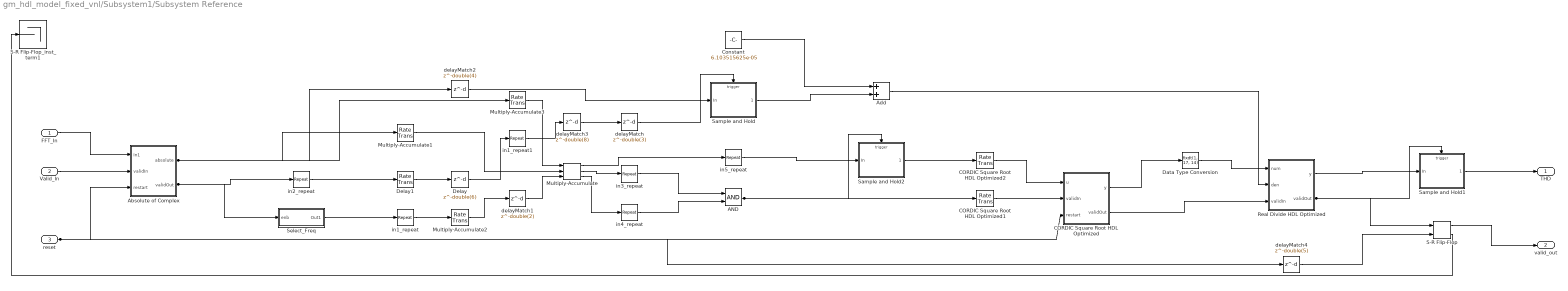
== system gm_hdl_model_fixed_vnl/Subsystem1/Subsystem Reference ==
  FFT_In : Inport  OutDataTypeStr=fixdt(1, 12, 11)  PortDimensions=[2]  SampleTime=1e-08
  Valid_In : Inport  Port=2  OutDataTypeStr=boolean  PortDimensions=1  SampleTime=1e-08
  reset : Inport  Port=3  OutDataTypeStr=boolean  PortDimensions=1  SampleTime=1e-08
  AND : Logic  AllPortsSameDT=off  OutDataTypeStr=boolean  SampleTime=5e-09
  Absolute of Complex : Subsystem
  Add : Sum  OutDataTypeStr=fixdt(1, 17, 14)  AccumDataTypeStr=fixdt(1, 17, 14)  SampleTime=5e-09
  CORDIC Square Root HDL Optimized : Subsystem  mask(CORDIC Square Root HDL Optimized){autoMaximumShiftVal=on, maximumShiftValue=double(10), nIterPerReg=double(1)}
      mask prompts: autoMaximumShiftVal "fixed:emblib:AutoCORDICMaxShiftValue"; maximumShiftValue "fixed:emblib:CORDICMaxShiftValue"; nIterPerReg "fixed:emblib:NumberOfIterationsPerReg"
      mask help: fixed:emblib:CORDICSquareRootHDLFullDescription
      mask Help: eval('embblk.embhelp(gcb)')
      mask Callback autoMaximumShiftVal:
      | autoMaxShiftVal = get_param(gcb,'autoMaximumShiftVal');
      | if strcmp(autoMaxShiftVal,'on')
      |     set_param(gcb,'MaskVisibilities',{'on','off','on'});
      | else
      |     set_param(gcb,'MaskVisibilities',{'on','on','on'});
      | end
      mask Display: disp('CORDIC Square Root\nHDL Optimized')
  CORDIC Square Root HDL Optimized1 : RateTransition  OutPortSampleTimeOpt=Multiple of input port sample time  OutPortSampleTimeMultiple=2
  CORDIC Square Root HDL Optimized2 : RateTransition  OutPortSampleTimeOpt=Multiple of input port sample time  OutPortSampleTimeMultiple=2
  Constant : Constant  Value=6.103515625e-05  OutDataTypeStr=fixdt(1, 16, 14)  SampleTime=5e-09
  Data Type Conversion : DataTypeConversion  OutDataTypeStr=fixdt(1, 17, 14)  SampleTime=1e-08  SaturateOnIntegerOverflow=off  RndMeth=Floor
  Delay : Delay  DelayLength=double(6)  InitialCondition=0  SampleTime=1e-08
  Delay1 : RateTransition  OutPortSampleTimeOpt=Multiple of input port sample time  OutPortSampleTimeMultiple=2
  Multiply-Accumulate : hdlsllib/HDL Operations/Multiply-Accumulate  opMode=Streaming - using Number of Samples  initValueSetting=Dialog  initValue=0  initValueSetting2=Dialog  initValue2=0  initValueSetting3=Dialog  initValue3=0  num_samples=1015  RndMeth2=Floor  RndMeth3=Floor  datatype2=Inherit: Inherit via back propagation  datatype3=fixdt(1, 22, 20)  validOut=on  endInandOut=on  startOut=on  countOut=off  dim=-1  DoSatur=off  parallel=off
  Multiply-Accumulate1 : RateTransition  OutPortSampleTimeOpt=Multiple of input port sample time  OutPortSampleTimeMultiple=2
  Multiply-Accumulate2 : RateTransition  OutPortSampleTimeOpt=Multiple of input port sample time  OutPortSampleTimeMultiple=2
  Multiply-Accumulate3 : RateTransition  OutPortSampleTimeOpt=Multiple of input port sample time  OutPortSampleTimeMultiple=2
  Real Divide HDL Optimized : Subsystem  mask(Real Divide HDL Optimized){OutputType=fixdt(1,18,10)}
      mask prompts: OutputType "fixed:emblib:OutputPrototype"
      mask help: fixed:emblib:RealDivideFullDescription
      mask Help: eval('embblk.embhelp(gcb)')
      mask Display:
      | text(0.5,0.6,'den ~= 0','texmode','on','HorizontalAlignment','center')
      | text(0.5,0.4,'y = num/den','texmode','on','HorizontalAlignment','center')
  S-R Flip-Flop : simulink_extras/Flip Flops/S-R Flip-Flop  initial_condition=0
  S-R Flip-Flop_inst_term1 : Terminator
  Sample and Hold : Subsystem  mask(Sample and Hold){trig=Rising edge, initCond=double(0), latchinput=off}
      mask prompts: trig "dsp:DSPSignalOperationsBlockDialog:TriggerType_MP"; initCond "dsp:DSPSignalOperationsBlockDialog:InitialCondition_MP"; latchinput "dsp:DSPSignalOperationsBlockDialog:LatchInput_MP"
      mask help: dsp:DSPSignalOperationsBlockDialog:SampleAndHold_MaskDesc
      mask init:
      | initCond = double(0);
      | latchinput = double(0);
      | s = 'rising';
      | trig = double(1);
      mask Help: eval('blocksethelp');
      mask TypeOptions trig: dsp:DSPSignalOperationsBlockDialog:RisingEdge_MP | dsp:DSPSignalOperationsBlockDialog:FallingEdge_MP | dsp:DSPSignalOperationsBlockDialog:EitherEdge_MP
      mask Display: disp('S/H')
  Sample and Hold1 : Subsystem  mask(Sample and Hold){trig=Rising edge, initCond=double(0), latchinput=off}
      mask prompts: trig "dsp:DSPSignalOperationsBlockDialog:TriggerType_MP"; initCond "dsp:DSPSignalOperationsBlockDialog:InitialCondition_MP"; latchinput "dsp:DSPSignalOperationsBlockDialog:LatchInput_MP"
      mask help: dsp:DSPSignalOperationsBlockDialog:SampleAndHold_MaskDesc
      mask init:
      | initCond = double(0);
      | latchinput = double(0);
      | s = 'rising';
      | trig = double(1);
      mask Help: eval('blocksethelp');
      mask TypeOptions trig: dsp:DSPSignalOperationsBlockDialog:RisingEdge_MP | dsp:DSPSignalOperationsBlockDialog:FallingEdge_MP | dsp:DSPSignalOperationsBlockDialog:EitherEdge_MP
      mask Display: disp('S/H')
  Sample and Hold2 : Subsystem  mask(Sample and Hold){trig=Rising edge, initCond=double(0), latchinput=off}
      mask prompts: trig "dsp:DSPSignalOperationsBlockDialog:TriggerType_MP"; initCond "dsp:DSPSignalOperationsBlockDialog:InitialCondition_MP"; latchinput "dsp:DSPSignalOperationsBlockDialog:LatchInput_MP"
      mask help: dsp:DSPSignalOperationsBlockDialog:SampleAndHold_MaskDesc
      mask init:
      | initCond = double(0);
      | latchinput = double(0);
      | s = 'rising';
      | trig = double(1);
      mask Help: eval('blocksethelp');
      mask TypeOptions trig: dsp:DSPSignalOperationsBlockDialog:RisingEdge_MP | dsp:DSPSignalOperationsBlockDialog:FallingEdge_MP | dsp:DSPSignalOperationsBlockDialog:EitherEdge_MP
      mask Display: disp('S/H')
  Select_Freq : Subsystem
  delayMatch : Delay  DelayLength=double(3)  InitialCondition=0  SampleTime=5e-09
  delayMatch1 : Delay  DelayLength=double(2)  InitialCondition=0  SampleTime=1e-08
  delayMatch2 : Delay  DelayLength=double(4)  InitialCondition=0  SampleTime=5e-09
  delayMatch3 : Delay  DelayLength=double(8)  InitialCondition=0  SampleTime=5e-09
  delayMatch4 : Delay  DelayLength=double(5)  InitialCondition=0  SampleTime=1e-08
  in1_repeat : dspsigops/Repeat  FactorSource=Dialog parameter  N=double(2)  Nmax=16  RateOptions=Allow multirate processing  ic=0  mode=Unused parameter value
  in1_repeat1 : dspsigops/Repeat  FactorSource=Dialog parameter  N=double(2)  Nmax=16  RateOptions=Allow multirate processing  ic=0  mode=Unused parameter value
  in2_repeat : dspsigops/Repeat  FactorSource=Dialog parameter  N=double(2)  Nmax=16  RateOptions=Allow multirate processing  ic=0  mode=Unused parameter value
  in3_repeat : dspsigops/Repeat  FactorSource=Dialog parameter  N=double(2)  Nmax=16  RateOptions=Allow multirate processing  ic=0  mode=Unused parameter value
  in4_repeat : dspsigops/Repeat  FactorSource=Dialog parameter  N=double(2)  Nmax=16  RateOptions=Allow multirate processing  ic=0  mode=Unused parameter value
  in5_repeat : dspsigops/Repeat  FactorSource=Dialog parameter  N=double(2)  Nmax=16  RateOptions=Allow multirate processing  ic=0  mode=Unused parameter value
  THD : Outport  SampleTime=1e-08
  valid_out : Outport  Port=2  SampleTime=1e-08
  wires:
  Sample and Hold/1(" ") -> Add/2
  delayMatch/1 -> Sample and Hold/Trigger
  reset/1 -> CORDIC Square Root HDL Optimized/3(restart), Absolute of Complex/3(restart), delayMatch4/1
  in1_repeat1/1 -> delayMatch3/1
  Absolute of Complex/1(absolute) -> Multiply-Accumulate1/1, Multiply-Accumulate3/1, delayMatch2/1
  Multiply-Accumulate2/1 -> delayMatch1/1
  Sample and Hold2/1(" ") -> CORDIC Square Root HDL Optimized2/1
  AND/1 -> Sample and Hold2/Trigger, CORDIC Square Root HDL Optimized1/1
  in5_repeat/1 -> Sample and Hold2/1(In)
  in4_repeat/1 -> AND/2
  in3_repeat/1 -> AND/1
  delayMatch3/1 -> delayMatch/1
  Constant/1 -> Add/1
  in2_repeat/1 -> Delay1/1
  in1_repeat/1 -> Multiply-Accumulate2/1
  Multiply-Accumulate3/1 -> Multiply-Accumulate/1
  Delay/1 -> in1_repeat1/1
  delayMatch1/1 -> Multiply-Accumulate/3
  Multiply-Accumulate1/1 -> Multiply-Accumulate/2
  Delay1/1 -> Delay/1
  delayMatch2/1 -> Sample and Hold/1(In)
  Add/1 -> Real Divide HDL Optimized/2(den)
  S-R Flip-Flop/2 -> S-R Flip-Flop_inst_term1/1
  Select_Freq/1(Out1) -> in1_repeat/1
  CORDIC Square Root HDL Optimized2/1 -> CORDIC Square Root HDL Optimized/1(u)
  Sample and Hold1/1(" ") -> THD/1
  S-R Flip-Flop/1 -> valid_out/1
  Real Divide HDL Optimized/2(validOut) -> S-R Flip-Flop/1, Sample and Hold1/Trigger
  Real Divide HDL Optimized/1(y) -> Sample and Hold1/1(In)
  Multiply-Accumulate/3 -> in4_repeat/1
  Multiply-Accumulate/2 -> in3_repeat/1
  Multiply-Accumulate/1 -> in5_repeat/1
  Data Type Conversion/1 -> Real Divide HDL Optimized/1(num)
  CORDIC Square Root HDL Optimized/2(validOut) -> Real Divide HDL Optimized/3(validIn)
  CORDIC Square Root HDL Optimized/1(y) -> Data Type Conversion/1
  Absolute of Complex/2(validOut) -> in2_repeat/1, Select_Freq/1(enb)
  CORDIC Square Root HDL Optimized1/1 -> CORDIC Square Root HDL Optimized/2(validIn)
  delayMatch4/1 -> S-R Flip-Flop/2
  Valid_In/1 -> Absolute of Complex/2(validIn)
  FFT_In/1 -> Absolute of Complex/1(In1)

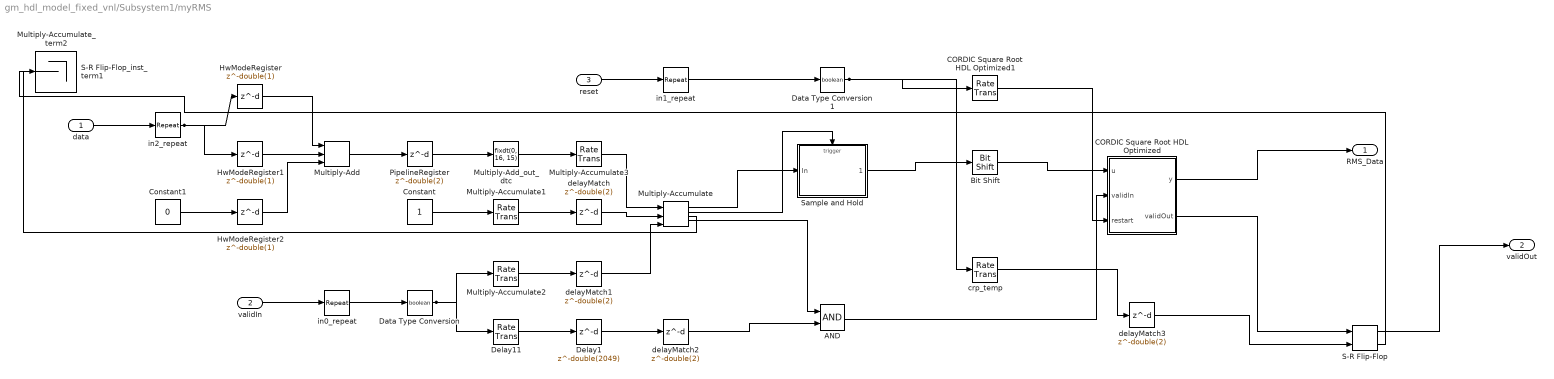
== system gm_hdl_model_fixed_vnl/Subsystem1/myRMS ==
  data : Inport  OutDataTypeStr=fixdt(1, 12, 11)  PortDimensions=1  SampleTime=1e-08
  validIn : Inport  Port=2  OutDataTypeStr=boolean  PortDimensions=1  SampleTime=1e-08
  reset : Inport  Port=3  OutDataTypeStr=boolean  PortDimensions=1  SampleTime=1e-08
  AND : Logic  AllPortsSameDT=off  OutDataTypeStr=boolean  SampleTime=1e-08
  Bit Shift : hdlsllib/Logic and Bit Operations/Bit Shift  mode=Shift Right Arithmetic  N=double(11)
  CORDIC Square Root HDL Optimized : Subsystem  mask(CORDIC Square Root HDL Optimized){autoMaximumShiftVal=on, maximumShiftValue=double(10), nIterPerReg=double(1)}
      mask prompts: autoMaximumShiftVal "fixed:emblib:AutoCORDICMaxShiftValue"; maximumShiftValue "fixed:emblib:CORDICMaxShiftValue"; nIterPerReg "fixed:emblib:NumberOfIterationsPerReg"
      mask help: fixed:emblib:CORDICSquareRootHDLFullDescription
      mask Help: eval('embblk.embhelp(gcb)')
      mask Callback autoMaximumShiftVal:
      | autoMaxShiftVal = get_param(gcb,'autoMaximumShiftVal');
      | if strcmp(autoMaxShiftVal,'on')
      |     set_param(gcb,'MaskVisibilities',{'on','off','on'});
      | else
      |     set_param(gcb,'MaskVisibilities',{'on','on','on'});
      | end
      mask Display: disp('CORDIC Square Root\nHDL Optimized')
  CORDIC Square Root HDL Optimized1 : RateTransition  OutPortSampleTimeOpt=Multiple of input port sample time  OutPortSampleTimeMultiple=2
  Constant : Constant  OutDataTypeStr=fixdt(0, 16, 15)  SampleTime=5e-09
  Constant1 : Constant  Value=0  OutDataTypeStr=fixdt(1, 12, 11)  SampleTime=5e-09
  Data Type Conversion : DataTypeConversion  OutDataTypeStr=boolean
  Data Type Conversion1 : DataTypeConversion  OutDataTypeStr=boolean
  Delay1 : Delay  DelayLength=double(2049)  InitialCondition=0  SampleTime=1e-08
  Delay11 : RateTransition  OutPortSampleTimeOpt=Multiple of input port sample time  OutPortSampleTimeMultiple=2
  HwModeRegister : Delay  DelayLength=double(1)  InitialCondition=0  SampleTime=5e-09
  HwModeRegister1 : Delay  DelayLength=double(1)  InitialCondition=0  SampleTime=5e-09
  HwModeRegister2 : Delay  DelayLength=double(1)  InitialCondition=0  SampleTime=5e-09
  Multiply-Accumulate : hdlsllib/HDL Operations/Multiply-Accumulate  opMode=Streaming - using Number of Samples  initValueSetting=Dialog  initValue=0  initValueSetting2=Dialog  initValue2=0  initValueSetting3=Dialog  initValue3=0  num_samples=2048  RndMeth2=Floor  RndMeth3=Floor  datatype2=Inherit: Inherit via back propagation  datatype3=fixdt(0, 16, 7)  validOut=on  endInandOut=on  startOut=on  countOut=on  dim=-1  DoSatur=off  parallel=off
  Multiply-Accumulate1 : RateTransition  OutPortSampleTimeOpt=Multiple of input port sample time  OutPortSampleTimeMultiple=2
  Multiply-Accumulate2 : RateTransition  OutPortSampleTimeOpt=Multiple of input port sample time  OutPortSampleTimeMultiple=2
  Multiply-Accumulate3 : RateTransition  OutPortSampleTimeOpt=Multiple of input port sample time  OutPortSampleTimeMultiple=2
  Multiply-Accumulate_term2 : Terminator
  Multiply-Add : hdlsllib/HDL Operations/Multiply-Add  Function=c+(a.*b)  datatype=fixdt(1, 25, 22)  DoSatur=off  FMA=off
  Multiply-Add_out_dtc : DataTypeConversion  OutDataTypeStr=fixdt(0, 16, 15)  SampleTime=5e-09  SaturateOnIntegerOverflow=off  RndMeth=Floor
  PipelineRegister : Delay  DelayLength=double(2)  InitialCondition=0  SampleTime=5e-09
  S-R Flip-Flop : simulink_extras/Flip Flops/S-R Flip-Flop  initial_condition=0
  S-R Flip-Flop_inst_term1 : Terminator
  Sample and Hold : Subsystem  mask(Sample and Hold){trig=Rising edge, initCond=double(0), latchinput=off}
      mask prompts: trig "dsp:DSPSignalOperationsBlockDialog:TriggerType_MP"; initCond "dsp:DSPSignalOperationsBlockDialog:InitialCondition_MP"; latchinput "dsp:DSPSignalOperationsBlockDialog:LatchInput_MP"
      mask help: dsp:DSPSignalOperationsBlockDialog:SampleAndHold_MaskDesc
      mask init:
      | initCond = double(0);
      | latchinput = double(0);
      | s = 'rising';
      | trig = double(1);
      mask Help: eval('blocksethelp');
      mask TypeOptions trig: dsp:DSPSignalOperationsBlockDialog:RisingEdge_MP | dsp:DSPSignalOperationsBlockDialog:FallingEdge_MP | dsp:DSPSignalOperationsBlockDialog:EitherEdge_MP
      mask Display: disp('S/H')
  crp_temp : RateTransition  OutPortSampleTimeOpt=Multiple of input port sample time  OutPortSampleTimeMultiple=2
  delayMatch{,1..3} (4 alike) : Delay  DelayLength=double(2)  InitialCondition=0  SampleTime=1e-08
  in0_repeat : dspsigops/Repeat  FactorSource=Dialog parameter  N=double(2)  Nmax=16  RateOptions=Allow multirate processing  ic=0  mode=Unused parameter value
  in1_repeat : dspsigops/Repeat  FactorSource=Dialog parameter  N=double(2)  Nmax=16  RateOptions=Allow multirate processing  ic=0  mode=Unused parameter value
  in2_repeat : dspsigops/Repeat  FactorSource=Dialog parameter  N=double(2)  Nmax=16  RateOptions=Allow multirate processing  ic=0  mode=Unused parameter value
  RMS_Data : Outport  SampleTime=1e-08
  validOut : Outport  Port=2  SampleTime=1e-08
  wires:
  HwModeRegister2/1 -> Multiply-Add/3
  HwModeRegister1/1 -> Multiply-Add/2
  HwModeRegister/1 -> Multiply-Add/1
  Multiply-Add/1 -> PipelineRegister/1
  PipelineRegister/1 -> Multiply-Add_out_dtc/1
  Constant1/1 -> HwModeRegister2/1
  crp_temp/1 -> delayMatch3/1
  Delay1/1 -> delayMatch2/1
  Multiply-Accumulate2/1 -> delayMatch1/1
  Multiply-Accumulate1/1 -> delayMatch/1
  Multiply-Add_out_dtc/1 -> Multiply-Accumulate3/1
  Data Type Conversion1/1 -> CORDIC Square Root HDL Optimized1/1, crp_temp/1
  Data Type Conversion/1 -> Multiply-Accumulate2/1, Delay11/1
  Constant/1 -> Multiply-Accumulate1/1
  in2_repeat/1 -> HwModeRegister1/1, HwModeRegister/1
  in1_repeat/1 -> Data Type Conversion1/1
  in0_repeat/1 -> Data Type Conversion/1
  Multiply-Accumulate3/1 -> Multiply-Accumulate/1
  delayMatch3/1 -> S-R Flip-Flop/2
  CORDIC Square Root HDL Optimized1/1 -> CORDIC Square Root HDL Optimized/3(restart)
  delayMatch2/1 -> AND/2
  delayMatch1/1 -> Multiply-Accumulate/3
  delayMatch/1 -> Multiply-Accumulate/2
  Delay11/1 -> Delay1/1
  S-R Flip-Flop/2 -> S-R Flip-Flop_inst_term1/1
  Sample and Hold/1(" ") -> Bit Shift/1
  S-R Flip-Flop/1 -> validOut/1
  Multiply-Accumulate/4 -> AND/1
  Multiply-Accumulate/3 -> Multiply-Accumulate_term2/1
  Multiply-Accumulate/2 -> Sample and Hold/Trigger
  Multiply-Accumulate/1 -> Sample and Hold/1(In)
  CORDIC Square Root HDL Optimized/2(validOut) -> S-R Flip-Flop/1
  CORDIC Square Root HDL Optimized/1(y) -> RMS_Data/1
  Bit Shift/1 -> CORDIC Square Root HDL Optimized/1(u)
  AND/1 -> CORDIC Square Root HDL Optimized/2(validIn)
  reset/1 -> in1_repeat/1
  validIn/1 -> in0_repeat/1
  data/1 -> in2_repeat/1

== system gm_hdl_model_fixed_vnl/Subsystem1/BUF_MIN_MAX_AVG/Sample and Hold1 ==
  In : Inport  OutDataTypeStr=fixdt(0, 16, 16)
  Trigger : TriggerPort  VariantControl=(inherit)  OutDataTypeStr=boolean
  " " : Outport  InitialOutput=0
  wires:
  In/1 -> " "/1

== system gm_hdl_model_fixed_vnl/Subsystem1/BUF_MIN_MAX_AVG/Sample and Hold2 ==
  In : Inport  OutDataTypeStr=fixdt(1, 16, 15)
  Trigger : TriggerPort  VariantControl=(inherit)  OutDataTypeStr=boolean
  " " : Outport  InitialOutput=0
  wires:
  In/1 -> " "/1
